simulink model "SimulinkEx"  (R2022b)
settings: Solver=VariableStepAuto  StartTime=0.0  StopTime=10.0  RelTol=1e-3
values from neighbouring files (symbols this model uses):
  fc1 = 3    [IntroductionSession.m]
settings Model: Creator=Orange  LastModifiedBy=Orange

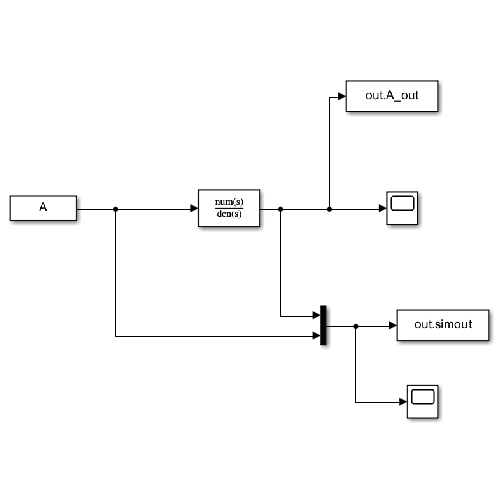
[thumbnail: Simulink's stored preview of the top-level diagram]
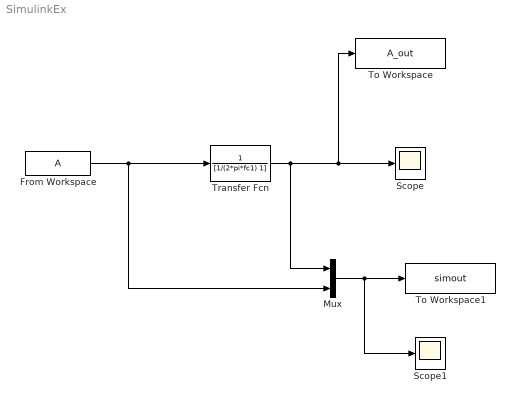
== system SimulinkEx ==
  From Workspace : FromWorkspace  VariableName=A
  Mux : Mux  Inputs=2
  Scope : Scope
  Scope1 : Scope
  To Workspace : ToWorkspace  VariableName=A_out  SampleTime=-1
  To Workspace1 : ToWorkspace  VariableName=simout  SampleTime=-1
  Transfer Fcn : TransferFcn  Denominator=[1/(2*pi*fc1) 1]
  wires:
  From Workspace/1 -> Mux/2, Transfer Fcn/1
  Transfer Fcn/1 -> Mux/1, To Workspace/1, Scope/1
  Mux/1 -> Scope1/1, To Workspace1/1
